simulink model "ARDroneHover"  (R2015b)
settings: Solver=VariableStepAuto  StartTime=0.0  StopTime=inf  RelTol=1e-3
values from neighbouring files (symbols this model uses):
  waypoints = getWaypoints()    [start.m]
undefined symbols (not defined in the file or in its folder): Angular, Linear
libraries: robotlib x4
settings Model: Creator=exbot  LastModifiedBy=exbot

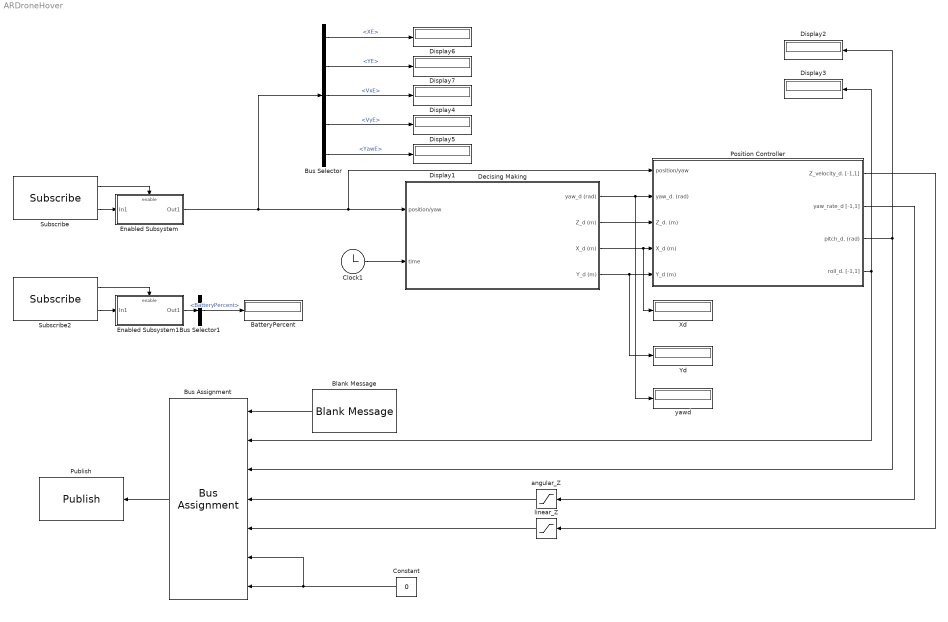
== system ARDroneHover ==
  BatteryPercent : Display
  Blank Message : robotlib/Blank Message  SourceLibraryInfo=This block requires Robotics System Toolbox  messageType=geometry_msgs/Twist  SampleTime=inf
  Bus Assignment : BusAssignment  AssignedSignals=Linear.Y,Linear.X,Angular.Z,Linear.Z,Angular.X,Angular.Y
  Bus Selector : BusSelector  OutputSignals=XE,YE,VxE,VyE,YawE
  Bus Selector1 : BusSelector  OutputSignals=BatteryPercent
  Clock1 : Clock
  Constant : Constant  Value=0
  Decising Making : Subsystem
  Display{1..7} (7 alike) : Display
  Enabled Subsystem : Subsystem  TreatAsAtomicUnit=on
  Enabled Subsystem1 : Subsystem  TreatAsAtomicUnit=on
  Position Controller : Subsystem  AncestorBlock=ARBlocks/Baseline Controller
  Publish : robotlib/Publish  SourceLibraryInfo=This block requires Robotics System Toolbox  topicSource=Select from ROS network  topic=/cmd_vel  messageType=geometry_msgs/Twist  messageQueueLength=1
  Subscribe : robotlib/Subscribe  SourceLibraryInfo=This block requires Robotics System Toolbox  topicSource=Select from ROS network  topic=/vpsnavdata  messageType=vps_driver/vps_navdata  sampleTime=-1  messageQueueLength=1
  Subscribe2 : robotlib/Subscribe  SourceLibraryInfo=This block requires Robotics System Toolbox  topicSource=Select from ROS network  topic=/ardrone/navdata  messageType=ardrone_autonomy/Navdata  sampleTime=-1  messageQueueLength=1
  Xd : Display
  Yd : Display
  angular_Z : Saturate  UpperLimit=0.1  LowerLimit=-0.1
  linear_Z : Saturate  UpperLimit=0.1  LowerLimit=-0.1
  yawd : Display
  wires:
  Decising Making/3(X_d (m)) -> Xd/1, Position Controller/4(X_d (m))
  Decising Making/4(Y_d (m)) -> Yd/1, Position Controller/5(Y_d (m))
  Decising Making/2(Z_d (m)) -> Position Controller/3(Z_d. (m))
  Enabled Subsystem1/1(Out1) -> Bus Selector1/1
  Bus Selector1/1 -> BatteryPercent/1  "<BatteryPercent>"
  Blank Message/1 -> Bus Assignment/1
  Position Controller/1(Z_velocity_d. [-1,1]) -> linear_Z/1
  Position Controller/2(yaw_rate_d [-1,1]) -> angular_Z/1
  Bus Assignment/1 -> Publish/1
  Subscribe/2 -> Enabled Subsystem/1(In1)
  Subscribe/1 -> Enabled Subsystem/Enable
  Subscribe2/2 -> Enabled Subsystem1/1(In1)
  Subscribe2/1 -> Enabled Subsystem1/Enable
  Constant/1 -> Bus Assignment/6, Bus Assignment/7
  Position Controller/4(roll_d. [-1,1]) -> Bus Assignment/2, Display3/1
  linear_Z/1 -> Bus Assignment/5
  angular_Z/1 -> Bus Assignment/4
  Position Controller/3(pitch_d. (rad)) -> Bus Assignment/3, Display2/1
  Decising Making/1(yaw_d (rad)) -> yawd/1, Position Controller/2(yaw_d. (rad))
  Bus Selector/1 -> Display6/1  "<XE>"
  Bus Selector/2 -> Display7/1  "<YE>"
  Bus Selector/3 -> Display4/1  "<VxE>"
  Bus Selector/4 -> Display5/1  "<VyE>"
  Enabled Subsystem/1(Out1) -> Bus Selector/1, Decising Making/1(position/yaw), Position Controller/1(" position/yaw ")
  Bus Selector/5 -> Display1/1  "<YawE>"
  Clock1/1 -> Decising Making/2(time)

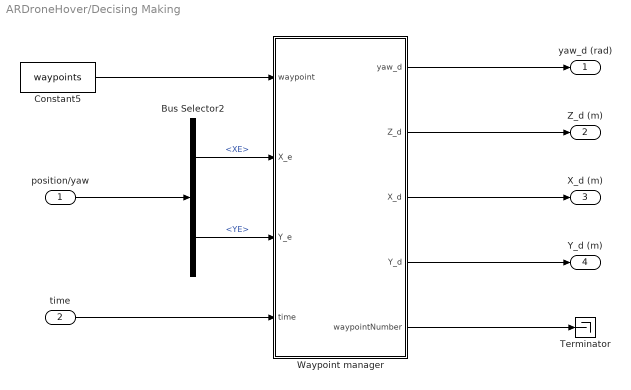
== system ARDroneHover/Decising Making ==
  position/yaw : Inport
  time : Inport  Port=2
  Bus Selector2 : BusSelector  OutputSignals=XE,YE
  Constant5 : Constant  Value=waypoints  VectorParams1D=off
  Terminator : Terminator
  "Waypoint manager " : MATLAB Function  TreatAsAtomicUnit=on
  yaw_d (rad) : Outport
  Z_d (m) : Outport  Port=2
  X_d (m) : Outport  Port=3
  Y_d (m) : Outport  Port=4
  wires:
  Bus Selector2/1 -> "Waypoint manager "/2(X_e)  "<XE>"
  Bus Selector2/2 -> "Waypoint manager "/3(Y_e)  "<YE>"
  position/yaw/1 -> Bus Selector2/1
  "Waypoint manager "/2(Z_d) -> Z_d (m)/1
  "Waypoint manager "/3(X_d) -> X_d (m)/1
  "Waypoint manager "/4(Y_d) -> Y_d (m)/1
  time/1 -> "Waypoint manager "/4(time)
  "Waypoint manager "/5(waypointNumber) -> Terminator/1
  "Waypoint manager "/1(yaw_d) -> yaw_d (rad)/1
  Constant5/1 -> "Waypoint manager "/1(waypoint)

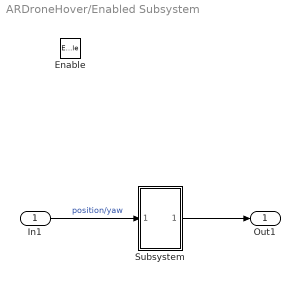
== system ARDroneHover/Enabled Subsystem ==
  In1 : Inport
  Enable : EnablePort
  Subsystem : Subsystem
  Out1 : Outport
  wires:
  In1/1 -> Subsystem/1(In1)  "position/yaw"
  Subsystem/1(Out1) -> Out1/1

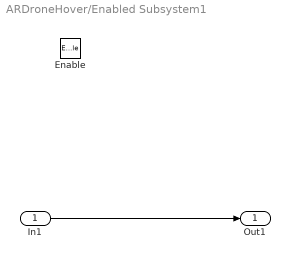
== system ARDroneHover/Enabled Subsystem1 ==
  In1 : Inport
  Enable : EnablePort
  Out1 : Outport
  wires:
  In1/1 -> Out1/1

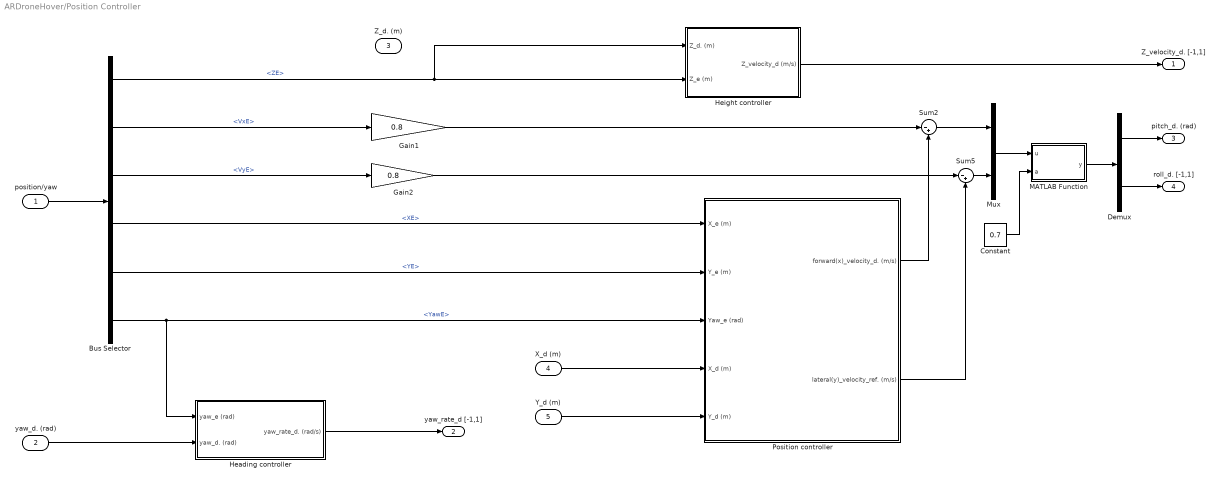
== system ARDroneHover/Position Controller ==
  " position/yaw " : Inport
  yaw_d. (rad) : Inport  Port=2
  Z_d. (m) : Inport  Port=3
  X_d (m) : Inport  Port=4
  Y_d (m) : Inport  Port=5
  Bus Selector : BusSelector  OutputSignals=ZE,VxE,VyE,XE,YE,YawE
  Constant : Constant  Value=0.7
  Demux : Demux  Outputs=2
  Gain1 : Gain  Gain=0.8
  Gain2 : Gain  Gain=0.8
  Heading controller : Subsystem
  "Height controller " : Subsystem
  MATLAB Function : MATLAB Function  TreatAsAtomicUnit=on
  Mux : Mux  Inputs=2
  Position controller : Subsystem
  Sum2 : Sum  Inputs=|-+
  Sum5 : Sum  Inputs=|-+
  Z_velocity_d. [-1,1] : Outport
  yaw_rate_d [-1,1] : Outport  Port=2
  pitch_d. (rad) : Outport  Port=3
  roll_d. [-1,1] : Outport  Port=4
  wires:
  Position controller/2(lateral(y)_velocity_ref. (m/s)) -> Sum5/2
  Gain2/1 -> Sum5/1
  Bus Selector/3 -> Gain2/1  "<VyE>"
  Position controller/1(forward(x)_velocity_d. (m/s)) -> Sum2/2
  Gain1/1 -> Sum2/1
  Bus Selector/6 -> Position controller/3(Yaw_e (rad)), Heading controller/1(yaw_e (rad))  "<YawE>"
  " position/yaw "/1 -> Bus Selector/1
  Bus Selector/1 -> "Height controller "/1(Z_d. (m)), "Height controller "/2(Z_e (m))  "<ZE>"
  "Height controller "/1(Z_velocity_d (m/s)) -> Z_velocity_d. [-1,1]/1
  Bus Selector/2 -> Gain1/1  "<VxE>"
  Heading controller/1(yaw_rate_d. (rad/s)) -> yaw_rate_d [-1,1]/1
  Bus Selector/4 -> Position controller/1(X_e (m))  "<XE>"
  Bus Selector/5 -> Position controller/2(Y_e (m))  "<YE>"
  X_d (m)/1 -> Position controller/4(X_d (m))
  Y_d (m)/1 -> Position controller/5(Y_d (m))
  Sum2/1 -> Mux/1
  Sum5/1 -> Mux/2
  yaw_d. (rad)/1 -> Heading controller/2(yaw_d. (rad))
  Mux/1 -> MATLAB Function/1(u)
  MATLAB Function/1(y) -> Demux/1
  Demux/1 -> pitch_d. (rad)/1
  Demux/2 -> roll_d. [-1,1]/1
  Constant/1 -> MATLAB Function/2(a)

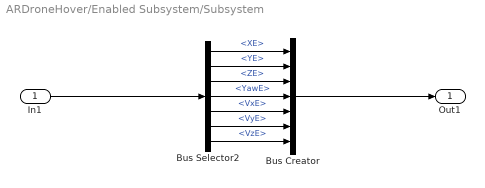
== system ARDroneHover/Enabled Subsystem/Subsystem ==
  In1 : Inport
  Bus Creator : BusCreator  Inputs=7
  Bus Selector2 : BusSelector  OutputSignals=XE,YE,ZE,YawE,VxE,VyE,VzE
  Out1 : Outport
  wires:
  Bus Creator/1 -> Out1/1
  Bus Selector2/2 -> Bus Creator/2  "<YE>"
  Bus Selector2/4 -> Bus Creator/4  "<YawE>"
  In1/1 -> Bus Selector2/1
  Bus Selector2/6 -> Bus Creator/6  "<VyE>"
  Bus Selector2/5 -> Bus Creator/5  "<VxE>"
  Bus Selector2/1 -> Bus Creator/1  "<XE>"
  Bus Selector2/3 -> Bus Creator/3  "<ZE>"
  Bus Selector2/7 -> Bus Creator/7  "<VzE>"

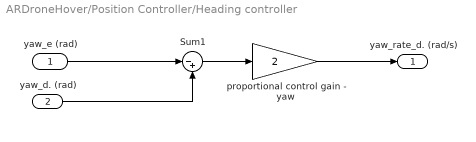
== system ARDroneHover/Position Controller/Heading controller ==
  yaw_e (rad) : Inport
  yaw_d. (rad) : Inport  Port=2
  Sum1 : Sum  Inputs=|-+
  proportional control gain - yaw : Gain  Gain=2
  yaw_rate_d. (rad/s) : Outport
  wires:
  Sum1/1 -> proportional control gain - yaw/1
  proportional control gain - yaw/1 -> yaw_rate_d. (rad/s)/1
  yaw_e (rad)/1 -> Sum1/1
  yaw_d. (rad)/1 -> Sum1/2

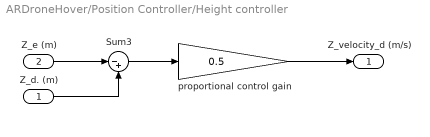
== system ARDroneHover/Position Controller/Height controller  ==
  Z_d. (m) : Inport
  Z_e (m) : Inport  Port=2
  Sum3 : Sum  Inputs=|-+
  proportional control gain : Gain  Gain=0.5
  Z_velocity_d (m/s) : Outport
  wires:
  proportional control gain/1 -> Z_velocity_d (m/s)/1
  Sum3/1 -> proportional control gain/1
  Z_e (m)/1 -> Sum3/1
  Z_d. (m)/1 -> Sum3/2

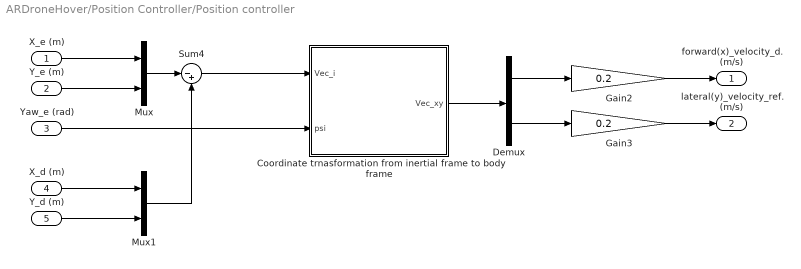
== system ARDroneHover/Position Controller/Position controller ==
  X_e (m) : Inport
  Y_e (m) : Inport  Port=2
  Yaw_e (rad) : Inport  Port=3
  X_d (m) : Inport  Port=4
  Y_d (m) : Inport  Port=5
  "Coordinate trnasformation from inertial frame to body frame " : MATLAB Function  TreatAsAtomicUnit=on
  Demux : Demux  Outputs=2
  Gain2 : Gain  Gain=0.2
  Gain3 : Gain  Gain=0.2
  Mux : Mux  Inputs=2
  Mux1 : Mux  Inputs=2
  Sum4 : Sum  Inputs=|-+
  forward(x)_velocity_d. (m/s) : Outport
  lateral(y)_velocity_ref. (m/s) : Outport  Port=2
  wires:
  Gain2/1 -> forward(x)_velocity_d. (m/s)/1
  Yaw_e (rad)/1 -> "Coordinate trnasformation from inertial frame to body frame "/2(psi)
  "Coordinate trnasformation from inertial frame to body frame "/1(Vec_xy) -> Demux/1
  Mux1/1 -> Sum4/2
  Sum4/1 -> "Coordinate trnasformation from inertial frame to body frame "/1(Vec_i)
  Y_e (m)/1 -> Mux/2
  X_e (m)/1 -> Mux/1
  Mux/1 -> Sum4/1
  X_d (m)/1 -> Mux1/1
  Y_d (m)/1 -> Mux1/2
  Demux/1 -> Gain2/1
  Demux/2 -> Gain3/1
  Gain3/1 -> lateral(y)_velocity_ref. (m/s)/1

== matlab function ARDroneHover/Position Controller/Position controller/Coordinate trnasformation from inertial frame to body frame  ==
  data: Vec_i input; Vec_xy output; psi input
function Vec_xy  = fcn(Vec_i , psi)
%#codegen
T = [cos(psi) sin(psi) ; -sin(psi) cos(psi)] ; 
Vec_xy = T*Vec_i(1:2,1);

== matlab function ARDroneHover/Position Controller/MATLAB Function ==
  data: u input; y output; a input
function y = fcn(u,a)
y = satgd(u,a);

== matlab function ARDroneHover/Decising Making/Waypoint manager  ==
  data: yaw_d output; Z_d output; waypoint input; X_e input; Y_e input; X_d output; Y_d output; time input; waypointNumber output
function [yaw_d, Z_d,  X_d, Y_d, waypointNumber]       = fcn(waypoint, X_e,Y_e, time )
nPoints = size(waypoint, 2) ;
persistent wpointer;
persistent t0 ;

if isempty(wpointer)
    wpointer = 1;
end

if isempty(t0)
    t0 = 0;
end

if ( norm([X_e,Y_e]' - waypoint(1:2, wpointer) )< 0.35) 
    yaw_d = waypoint(4, wpointer) ; % 当飞机进入目标航路点时，
                                                                   % 开始把当前航路点的期望偏航角赋值给控制器，
                                                                   % 控制机头指向下一个航路点
    if(wpointer ~= nPoints)        
        if (t0 ==0)
            t0 = time;
        else
            if ((time - t0 > waypoint(5, wpointer)))  % 严格来说飞机在当前航路点的悬停时间
                                                                                   % 应该要足以把偏航角控制到位
                                                                                   % 或者在判断语句中加入偏航角控制到位的判断
                 if(wpointer < nPoints)
                    wpointer = wpointer+ 1;
                    t0 = 0;
                 end                                           
            end
        end         
    end    
else  % 如果飞机离开当前航路点，飞向下一个航路点，
          % 应该继续把当前航路点的期望偏航角赋值给控制器，
          % 因为飞机需要在飞行过程中继续指向下一个航路点
    if(wpointer>1)
        yaw_d = waypoint(4, wpointer-1) ;
    else
        yaw_d = 0;
    end
end
%% Outputs
Z_d =  waypoint(3, wpointer) ;
X_d = waypoint(1, wpointer) ;
Y_d = waypoint(2, wpointer) ;
waypointNumber = wpointer ;
